simulink model "Jeos6DOF_IMU"  (R2022b)
settings: Solver=ode4  StartTime=0.0  StopTime=100  FixedStep=0.1  RelTol=1e-3
values from neighbouring files (symbols this model uses):
  a0_s2 = 0    [computeAeroForces.m]
  a0_s3 = 0    [computeAeroForces.m]
  a0_s4 = 0.05    [computeAeroForces.m]
  a0_s5 = 0.05    [computeAeroForces.m]
  AR_s2 = b_s2/c_s2    [computeSurfacePos.m]
  AR_s3 = b_s3/c_s3    [computeSurfacePos.m]
  AR_s4 = (b_s4 + b_s5)/c_s4    [computeSurfacePos.m]
  AR_s5 = (b_s4 + b_s5)/c_s5    [computeSurfacePos.m]
  area_s2 = c_s2 * b_s2    [computeSurfacePos.m]
  area_s3 = c_s3 * b_s3    [computeSurfacePos.m]
  area_s4 = c_s4 * b_s4    [computeSurfacePos.m]
  area_s5 = c_s5 * b_s5    [computeSurfacePos.m]
  c_s2 = componentMassesAndGeom(3,2)    [computeSurfacePos.m]
  c_s3 = componentMassesAndGeom(4,2)    [computeSurfacePos.m]
  c_s4 = componentMassesAndGeom(1,2)    [computeSurfacePos.m]
  c_s5 = componentMassesAndGeom(2,2)    [computeSurfacePos.m]
  CD0_s2 = 0.01    [computeAeroForces.m]
  CD0_s3 = 0.01    [computeAeroForces.m]
  CD0_s4 = 0.01    [computeAeroForces.m]
  CD0_s5 = 0.01    [computeAeroForces.m]
  CDa_s2 = 1    [computeAeroForces.m]
  CDa_s3 = 1    [computeAeroForces.m]
  CDa_s4 = 1    [computeAeroForces.m]
  CDa_s5 = 1    [computeAeroForces.m]
  CL0_s2 = 0    [computeAeroForces.m]
  CL0_s3 = 0    [computeAeroForces.m]
  CL0_s4 = 0.05    [computeAeroForces.m]
  CL0_s5 = 0.05    [computeAeroForces.m]
  CM0_s2 = 0    [computeAeroForces.m]
  CM0_s3 = 0    [computeAeroForces.m]
  CM0_s4 = -0.05    [computeAeroForces.m]
  CM0_s5 = -0.05    [computeAeroForces.m]
  CMa_s2 = 0    [computeAeroForces.m]
  CMa_s3 = 0    [computeAeroForces.m]
  CMa_s4 = 0    [computeAeroForces.m]
  CMa_s5 = 0    [computeAeroForces.m]
  e_s2 = 0.8    [computeAeroForces.m]
  e_s3 = 0.8    [computeAeroForces.m]
  e_s4 = 0.9    [computeAeroForces.m]
  e_s5 = 0.9    [computeAeroForces.m]
  i_s2 = 0    [computeAeroForces.m]
  i_s3 = 0    [computeAeroForces.m]
  i_s4 = 0.05    [computeAeroForces.m]
  i_s5 = 0.05    [computeAeroForces.m]
  Jxx = 1    [Sim_sixDOFdriverScript.m]
  Jxy = 0.    (= 0)    [Sim_sixDOFdriverScript.m]
  Jxz = 3    [Sim_sixDOFdriverScript.m]
  Jyx = 2    [Sim_sixDOFdriverScript.m]
  Jyy = 2    [Sim_sixDOFdriverScript.m]
  Jyz = 0    [Sim_sixDOFdriverScript.m]
  Jzx = Jxz    (= 3)    [Sim_sixDOFdriverScript.m]
  Jzy = Jyz    (= 0)    [Sim_sixDOFdriverScript.m]
  Jzz = 2    [Sim_sixDOFdriverScript.m]
  LL = 0.8    [Sim_sixDOFdriverScript.m]
  MM = 0.8    [Sim_sixDOFdriverScript.m]
  n_s2 = [0; 0; -1]    [computeAeroForces.m]
  n_s3 = [0; 1; 0]    [computeAeroForces.m]
  n_s4 = [0; 0; -1]    [computeAeroForces.m]
  n_s5 = [0; 0; -1]    [computeAeroForces.m]
  NN = 0.8    [Sim_sixDOFdriverScript.m]
  rEarth = 6378100    [Sim_sixDOFdriverScript.m]
  ro = 1.225    [computeAeroForces.m]
  x_S2_B_B = (x_S2_B_B_nominal + [0.25*c_s2 0 0]') - x_cg    [computeMassProps.m]
  x_S3_B_B = (x_S3_B_B_nominal + [0.25*c_s3 0 0]') - x_cg    [computeMassProps.m]
  x_S4_B_B = (x_S4_B_B_nominal + [0.25*c_s4 0 0]') - x_cg    [computeMassProps.m]
  x_S5_B_B = (x_S5_B_B_nominal + [0.25*c_s5 0 0]') - x_cg    [computeMassProps.m]
undefined symbols (not defined in the file or in its folder): earthRadius
libraries: simulink_extras x4, matrix_library x3, aerolibutil x2, sharedutil x1, simulink x1
(part 1 of 2)
settings Model: Creator=Jeo  LastModifiedBy=Jeo

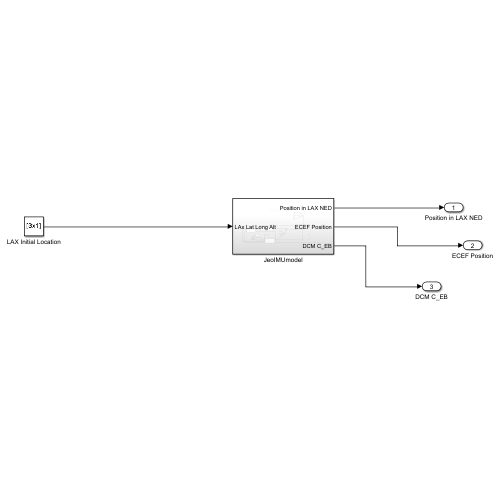
[thumbnail: Simulink's stored preview of the top-level diagram]
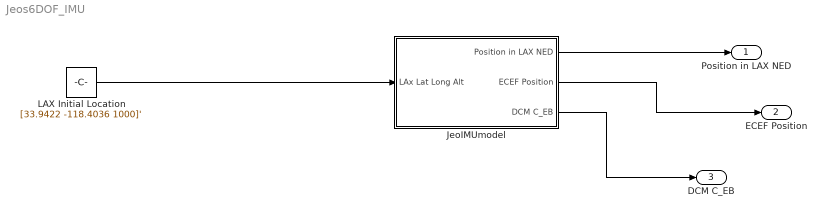
== system Jeos6DOF_IMU ==
  JeoIMUmodel : Subsystem
  LAX Initial Location : Constant  Value=[33.9422 -118.4036 1000]'
  Position in LAX NED : Outport
  ECEF Position : Outport  Port=2
  DCM C_EB : Outport  Port=3
  wires:
  LAX Initial Location/1 -> JeoIMUmodel/1(LAx Lat Long Alt)
  JeoIMUmodel/1(Position in LAX NED) -> Position in LAX NED/1
  JeoIMUmodel/2(ECEF Position) -> ECEF Position/1
  JeoIMUmodel/3(DCM C_EB) -> DCM C_EB/1

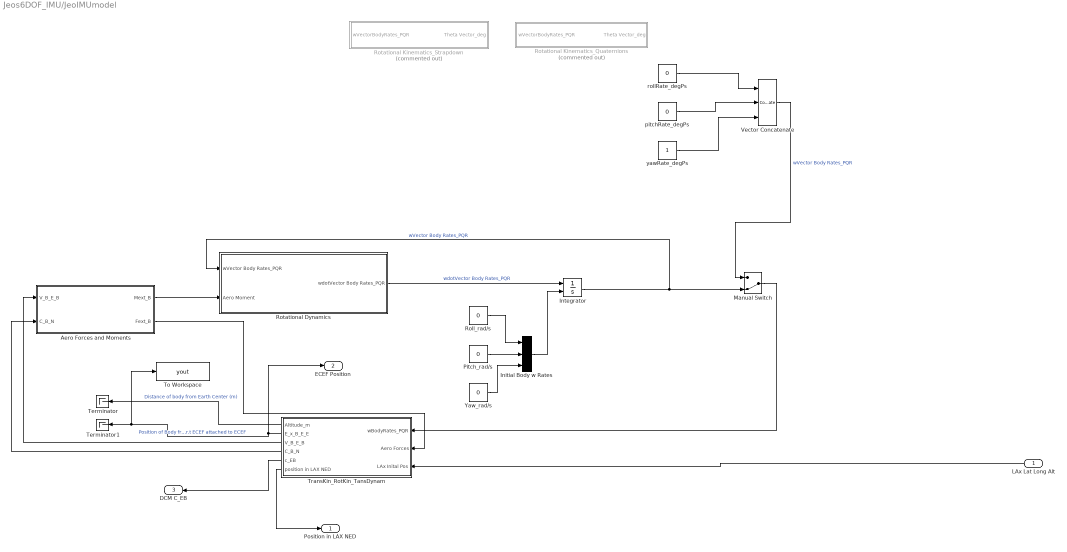
== system Jeos6DOF_IMU/JeoIMUmodel ==
  LAx Lat Long Alt : Inport
  Aero Forces and Moments : Subsystem
  Initial Body w Rates : Concatenate  NumInputs=3
  Integrator : Integrator  InitialConditionSource=external
  Manual Switch : ManualSwitch  CurrentSetting=0
  Pitch_rad/s : Constant  Value=0
  Roll_rad/s : Constant  Value=0
  Rotational Dynamics : Subsystem
  Rotational Kinematics_Quaternions : Subsystem  Commented=on
  Rotational Kinematics_Strapdown : Subsystem  Commented=on
  Terminator : Terminator
  Terminator1 : Terminator
  To Workspace : ToWorkspace  VariableName=yout  SaveFormat=Timeseries  SampleTime=-1
  TransKin_RotKin_TansDynam : Subsystem
  Vector Concatenate : Concatenate  NumInputs=3  Mode=Multidimensional array
  Yaw_rad/s : Constant  Value=0
  pitchRate_degPs : Constant  Value=0
  rollRate_degPs : Constant  Value=0
  yawRate_degPs : Constant
  Position in LAX NED : Outport
  ECEF Position : Outport  Port=2
  DCM C_EB : Outport  Port=3
  wires:
  TransKin_RotKin_TansDynam/2(E_x_B_E_E) -> Terminator1/1, To Workspace/1, ECEF Position/1  "Position of Body from ECEF w.r.t ECEF attached to ECEF"
  TransKin_RotKin_TansDynam/3(V_B_E_B) -> Aero Forces and Moments/1(V_B_E_B)
  Manual Switch/1 -> TransKin_RotKin_TansDynam/1(wBodyRates_PQR)
  TransKin_RotKin_TansDynam/1(Altitude_m) -> Terminator/1  "Distance of body from Earth Center (m)"
  Rotational Dynamics/1(wdotVector Body Rates_PQR) -> Integrator/1  "wdotVector Body Rates_PQR"
  Vector Concatenate/1 -> Manual Switch/1  "wVector Body Rates_PQR"
  TransKin_RotKin_TansDynam/4(C_B_N) -> Aero Forces and Moments/2(C_B_N)
  Integrator/1 -> Manual Switch/2, Rotational Dynamics/1(wVector Body Rates_PQR)  "wVector Body Rates_PQR"
  yawRate_degPs/1 -> Vector Concatenate/3
  Initial Body w Rates/1 -> Integrator/2
  Pitch_rad/s/1 -> Initial Body w Rates/2
  Aero Forces and Moments/1(Mext_B) -> Rotational Dynamics/2(Aero Moment)
  LAx Lat Long Alt/1 -> TransKin_RotKin_TansDynam/3(LAx Inital Pos)
  Roll_rad/s/1 -> Initial Body w Rates/1
  Aero Forces and Moments/2(Fext_B) -> TransKin_RotKin_TansDynam/2(Aero Forces)
  Yaw_rad/s/1 -> Initial Body w Rates/3
  rollRate_degPs/1 -> Vector Concatenate/1
  pitchRate_degPs/1 -> Vector Concatenate/2
  TransKin_RotKin_TansDynam/5(c_EB) -> DCM C_EB/1
  TransKin_RotKin_TansDynam/6(position in LAX NED) -> Position in LAX NED/1

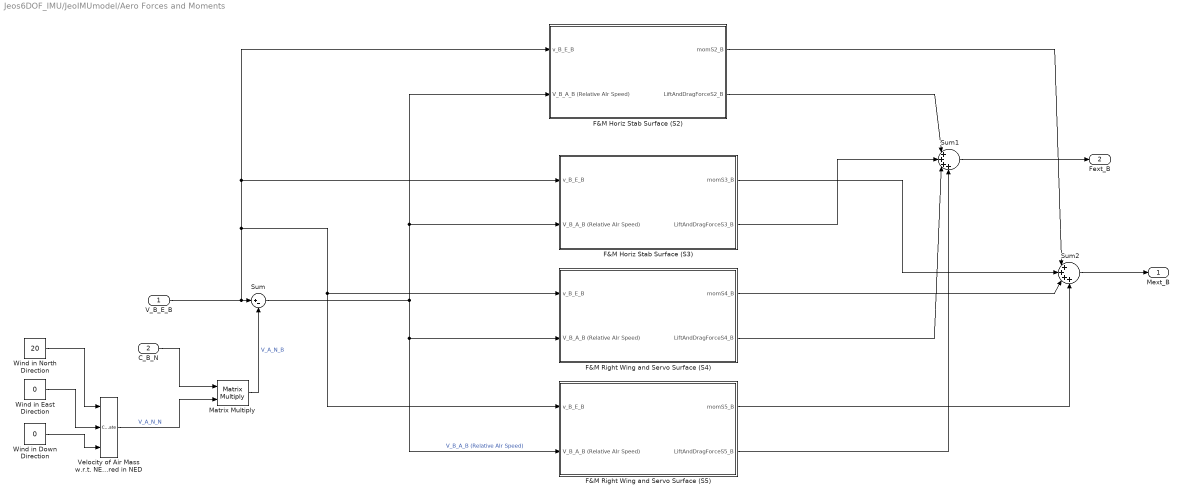
== system Jeos6DOF_IMU/JeoIMUmodel/Aero Forces and Moments ==
  V_B_E_B : Inport
  C_B_N : Inport  Port=2
  F&M Horiz Stab Surface (S2) : Subsystem
  F&M Horiz Stab Surface (S3) : Subsystem
  F&M Right Wing and Servo Surface (S4) : Subsystem
  F&M Right Wing and Servo Surface (S5) : Subsystem
  Matrix Multiply : Product  Multiplication=Matrix(*)
  Sum : Sum  Inputs=|+-
  Sum1 : Sum  Inputs=|++++
  Sum2 : Sum  Inputs=|++++
  Velocity of Air Mass w.r.t. NED as measured in NED : Concatenate  NumInputs=3
  Wind in Down Direction : Constant  Value=0
  Wind in East Direction : Constant  Value=0
  Wind in North Direction : Constant  Value=20
  Mext_B : Outport
  Fext_B : Outport  Port=2
  wires:
  V_B_E_B/1 -> F&M Right Wing and Servo Surface (S5)/1(v_B_E_B), F&M Right Wing and Servo Surface (S4)/1(v_B_E_B), F&M Horiz Stab Surface (S2)/1(v_B_E_B), F&M Horiz Stab Surface (S3)/1(v_B_E_B), Sum/1
  Velocity of Air Mass w.r.t. NED as measured in NED/1 -> Matrix Multiply/2  "V_A_N_N"
  Wind in North Direction/1 -> Velocity of Air Mass w.r.t. NED as measured in NED/1
  Wind in East Direction/1 -> Velocity of Air Mass w.r.t. NED as measured in NED/2
  Wind in Down Direction/1 -> Velocity of Air Mass w.r.t. NED as measured in NED/3
  Sum/1 -> F&M Horiz Stab Surface (S2)/2(V_B_A_B (Relative AIr Speed)), F&M Horiz Stab Surface (S3)/2(V_B_A_B (Relative AIr Speed)), F&M Right Wing and Servo Surface (S5)/2(V_B_A_B (Relative AIr Speed)), F&M Right Wing and Servo Surface (S4)/2(V_B_A_B (Relative AIr Speed))  "V_B_A_B (Relative AIr Speed)"
  F&M Horiz Stab Surface (S2)/2(LiftAndDragForceS2_B) -> Sum1/1
  F&M Horiz Stab Surface (S3)/2(LiftAndDragForceS3_B) -> Sum1/2
  F&M Right Wing and Servo Surface (S4)/2(LiftAndDragForceS4_B) -> Sum1/3
  F&M Right Wing and Servo Surface (S5)/2(LiftAndDragForceS5_B) -> Sum1/4
  Sum1/1 -> Fext_B/1
  F&M Horiz Stab Surface (S2)/1(momS2_B) -> Sum2/1
  F&M Horiz Stab Surface (S3)/1(momS3_B) -> Sum2/2
  F&M Right Wing and Servo Surface (S4)/1(momS4_B) -> Sum2/3
  F&M Right Wing and Servo Surface (S5)/1(momS5_B) -> Sum2/4
  Sum2/1 -> Mext_B/1
  C_B_N/1 -> Matrix Multiply/1
  Matrix Multiply/1 -> Sum/2  "V_A_N_B"

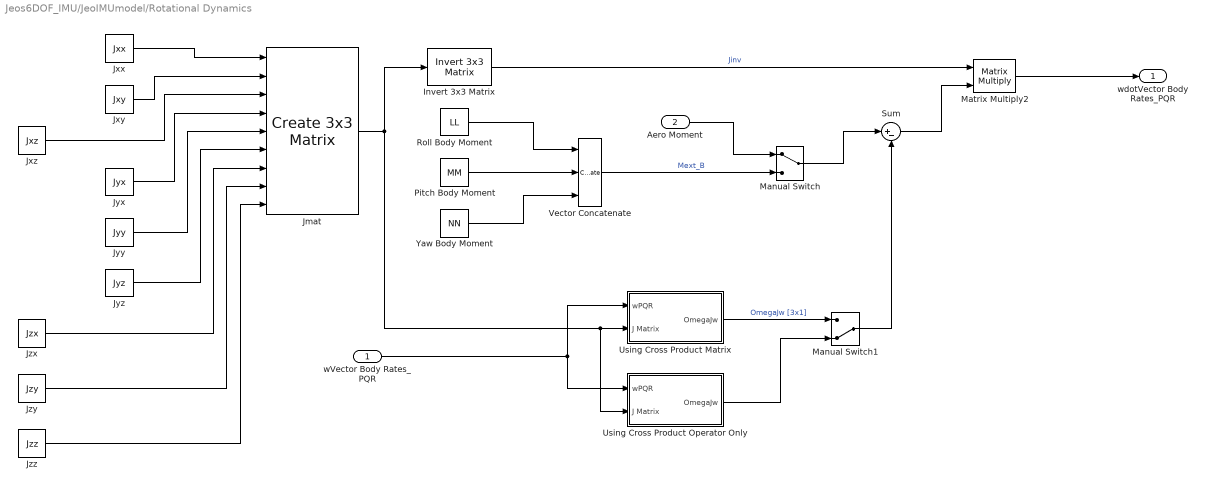
== system Jeos6DOF_IMU/JeoIMUmodel/Rotational Dynamics ==
  wVector Body Rates_PQR : Inport
  Aero Moment : Inport  Port=2
  Invert 3x3 Matrix : aerolibutil/Invert  3x3 Matrix
  Jmat : sharedutil/Create 3x3 Matrix  aMode=aMode
      settings: LibrarySourceBlock=aerolibutil/Create 3x3 Matrix
  Jxx : Constant  Value=Jxx
  Jxy : Constant  Value=Jxy
  Jxz : Constant  Value=Jxz
  Jyx : Constant  Value=Jyx
  Jyy : Constant  Value=Jyy
  Jyz : Constant  Value=Jyz
  Jzx : Constant  Value=Jzx
  Jzy : Constant  Value=Jzy
  Jzz : Constant  Value=Jzz
  Manual Switch : ManualSwitch
  Manual Switch1 : ManualSwitch  CurrentSetting=0
  Matrix Multiply2 : Product  Multiplication=Matrix(*)
  Pitch Body Moment : Constant  Value=MM
  Roll Body Moment : Constant  Value=LL
  Sum : Sum  Inputs=|+-
  Using Cross Product Matrix : Subsystem
  Using Cross Product Operator Only : Subsystem
  Vector Concatenate : Concatenate  NumInputs=3
  Yaw Body Moment : Constant  Value=NN
  wdotVector Body Rates_PQR : Outport
  wires:
  wVector Body Rates_PQR/1 -> Using Cross Product Operator Only/1(wPQR), Using Cross Product Matrix/1(wPQR)
  Jmat/1 -> Using Cross Product Matrix/2(J Matrix), Using Cross Product Operator Only/2(J Matrix), Invert 3x3 Matrix/1
  Using Cross Product Matrix/1(OmegaJw) -> Manual Switch1/1  "OmegaJw [3x1]"
  Sum/1 -> Matrix Multiply2/2
  Matrix Multiply2/1 -> wdotVector Body Rates_PQR/1
  Jxx/1 -> Jmat/1
  Jxy/1 -> Jmat/2
  Jxz/1 -> Jmat/3
  Jyx/1 -> Jmat/4
  Jyy/1 -> Jmat/5
  Jyz/1 -> Jmat/6
  Jzx/1 -> Jmat/7
  Jzy/1 -> Jmat/8
  Jzz/1 -> Jmat/9
  Invert 3x3 Matrix/1 -> Matrix Multiply2/1  "Jinv"
  Roll Body Moment/1 -> Vector Concatenate/1
  Pitch Body Moment/1 -> Vector Concatenate/2
  Yaw Body Moment/1 -> Vector Concatenate/3
  Vector Concatenate/1 -> Manual Switch/2  "Mext_B"
  Aero Moment/1 -> Manual Switch/1
  Manual Switch/1 -> Sum/1
  Manual Switch1/1 -> Sum/2
  Using Cross Product Operator Only/1(OmegaJw) -> Manual Switch1/2

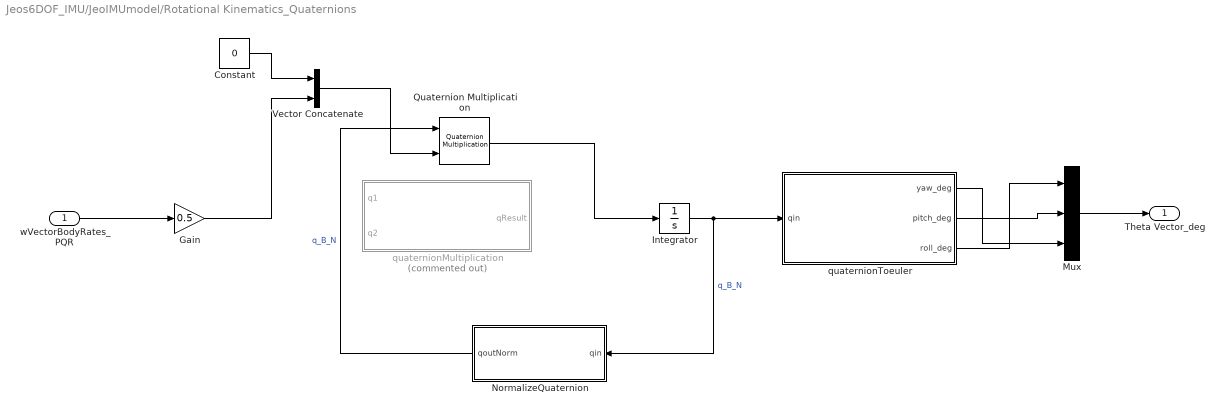
== system Jeos6DOF_IMU/JeoIMUmodel/Rotational Kinematics_Quaternions ==
  wVectorBodyRates_PQR : Inport
  Constant : Constant  Value=0
  Gain : Gain  Gain=0.5
  Integrator : Integrator
  Mux : Mux  Inputs=3
  NormalizeQuaternion : MATLAB Function  TreatAsAtomicUnit=on
  Quaternion Multiplication : aerolibutil/Quaternion Multiplication
  Vector Concatenate : Concatenate
  quaternionMultiplication : MATLAB Function  Commented=on  TreatAsAtomicUnit=on
  quaternionToeuler : MATLAB Function  TreatAsAtomicUnit=on
  Theta Vector_deg : Outport
  wires:
  wVectorBodyRates_PQR/1 -> Gain/1
  Gain/1 -> Vector Concatenate/2
  Constant/1 -> Vector Concatenate/1
  Integrator/1 -> NormalizeQuaternion/1(qin), quaternionToeuler/1(qin)  "q_B_N"
  quaternionToeuler/3(roll_deg) -> Mux/1
  quaternionToeuler/2(pitch_deg) -> Mux/2
  quaternionToeuler/1(yaw_deg) -> Mux/3
  NormalizeQuaternion/1(qoutNorm) -> Quaternion Multiplication/1  "q_B_N"
  Mux/1 -> Theta Vector_deg/1
  Quaternion Multiplication/1 -> Integrator/1
  Vector Concatenate/1 -> Quaternion Multiplication/2

== system Jeos6DOF_IMU/JeoIMUmodel/Rotational Kinematics_Strapdown ==
  wVectorBodyRates_PQR : Inport
  Demux : Demux  Outputs=3
  Integrator : Integrator
  MatrixMultiply : Product  Multiplication=Matrix(*)
  Mux : Mux  Inputs=3
  Omega_B_N : MATLAB Function  TreatAsAtomicUnit=on
  dcmTOeuler : MATLAB Function  TreatAsAtomicUnit=on
  Theta Vector_deg : Outport
  wires:
  wVectorBodyRates_PQR/1 -> Demux/1
  Demux/1 -> Omega_B_N/1(P_degPs)
  Demux/2 -> Omega_B_N/2(Q_degPs)
  Demux/3 -> Omega_B_N/3(R_degPs)
  Omega_B_N/1(y) -> MatrixMultiply/1  "omega_B_N"
  MatrixMultiply/1 -> Integrator/1  "cdot_N_B"
  Integrator/1 -> MatrixMultiply/2, dcmTOeuler/1(inputDCM)  "c_N_B"
  dcmTOeuler/3(roll_deg) -> Mux/1
  dcmTOeuler/2(pitch_deg) -> Mux/2
  dcmTOeuler/1(yaw_deg) -> Mux/3
  Mux/1 -> Theta Vector_deg/1  "Theta Vector_deg"

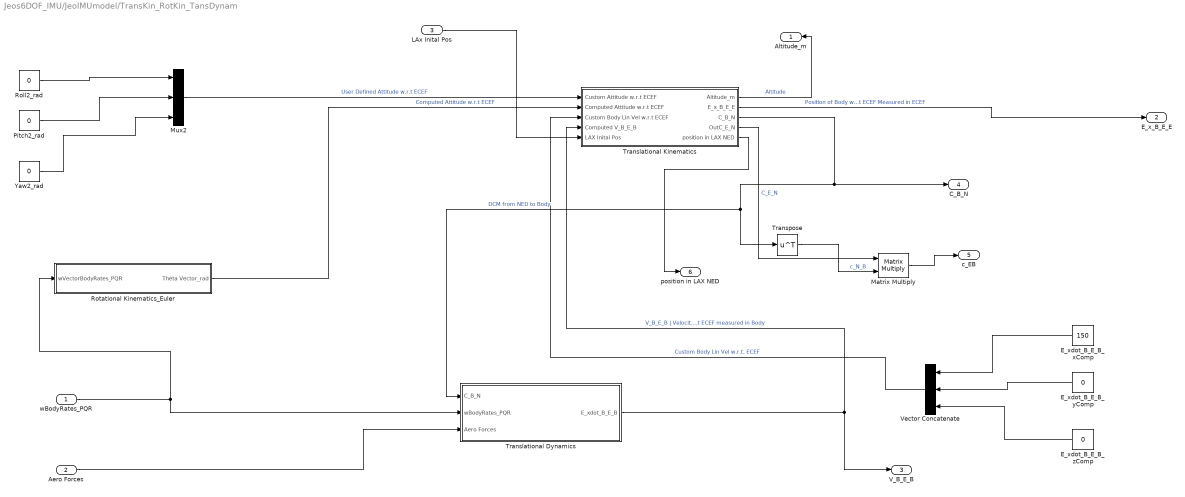
== system Jeos6DOF_IMU/JeoIMUmodel/TransKin_RotKin_TansDynam ==
  wBodyRates_PQR : Inport
  Aero Forces : Inport  Port=2
  LAx Inital Pos : Inport  Port=3
  E_xdot_B_E_B_xComp : Constant  Value=150
  E_xdot_B_E_B_yComp : Constant  Value=0
  E_xdot_B_E_B_zComp : Constant  Value=0
  Matrix Multiply : Product  Multiplication=Matrix(*)
  Mux2 : Mux  Inputs=3
  Pitch2_rad : Constant  Value=0
  Roll2_rad : Constant  Value=0
  Rotational Kinematics_Euler : Subsystem
  Translational Dynamics : Subsystem
  Translational Kinematics : Subsystem
  Transpose : Math  Operator=transpose
  Vector Concatenate : Concatenate  NumInputs=3
  Yaw2_rad : Constant  Value=0
  Altitude_m : Outport
  E_x_B_E_E : Outport  Port=2
  V_B_E_B : Outport  Port=3
  C_B_N : Outport  Port=4
  c_EB : Outport  Port=5
  position in LAX NED : Outport  Port=6
  wires:
  Pitch2_rad/1 -> Mux2/2
  Translational Dynamics/1(E_xdot_B_E_B) -> Translational Kinematics/4(Computed V_B_E_B), V_B_E_B/1  "V_B_E_B | Velocity of Body w.r.t ECEF measured in Body"
  wBodyRates_PQR/1 -> Translational Dynamics/2(wBodyRates_PQR), Rotational Kinematics_Euler/1(wVectorBodyRates_PQR)
  Roll2_rad/1 -> Mux2/1
  Yaw2_rad/1 -> Mux2/3
  E_xdot_B_E_B_xComp/1 -> Vector Concatenate/1
  E_xdot_B_E_B_yComp/1 -> Vector Concatenate/2
  E_xdot_B_E_B_zComp/1 -> Vector Concatenate/3
  Aero Forces/1 -> Translational Dynamics/3(Aero Forces)
  Mux2/1 -> Translational Kinematics/1(Custom Attitude w.r.t ECEF)  "User Defined Attitude w.r.t ECEF"
  Rotational Kinematics_Euler/1(Theta Vector_rad) -> Translational Kinematics/2(Computed Attitude w.r.t ECEF)  "Computed Attitude w.r.t ECEF"
  Vector Concatenate/1 -> Translational Kinematics/3(Custom Body Lin Vel w.r.t ECEF)  "Custom Body Lin Vel w.r.t. ECEF"
  Translational Kinematics/1(Altitude_m) -> Altitude_m/1  "Altitude"
  Translational Kinematics/2(E_x_B_E_E) -> E_x_B_E_E/1  "Position of Body w.r.t ECEF Measured in ECEF"
  Translational Kinematics/3(C_B_N) -> Transpose/1, Translational Dynamics/1(C_B_N), C_B_N/1  "DCM from NED to Body"
  LAx Inital Pos/1 -> Translational Kinematics/5(LAX Inital Pos)
  Matrix Multiply/1 -> c_EB/1
  Transpose/1 -> Matrix Multiply/2  "c_N_B"
  Translational Kinematics/4(OutC_E_N) -> Matrix Multiply/1  "C_E_N"
  Translational Kinematics/5(position in LAX NED) -> position in LAX NED/1

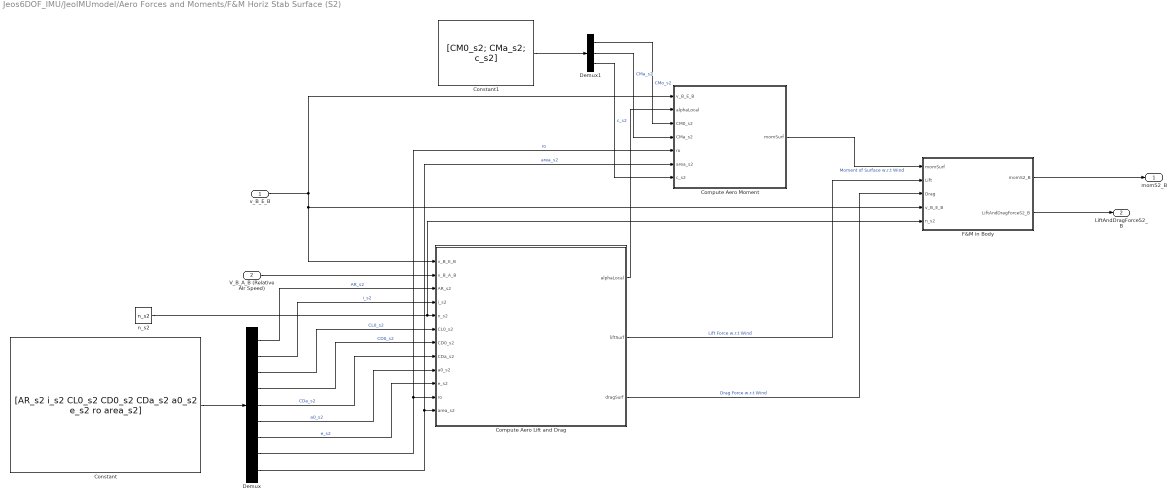
== system Jeos6DOF_IMU/JeoIMUmodel/Aero Forces and Moments/F&M Horiz Stab Surface (S2) ==
  v_B_E_B : Inport
  V_B_A_B (Relative AIr Speed) : Inport  Port=2
  Compute Aero Lift and Drag : MATLAB Function  TreatAsAtomicUnit=on
  Compute Aero Moment : MATLAB Function  TreatAsAtomicUnit=on
  Constant : Constant  Value=[AR_s2 i_s2 CL0_s2 CD0_s2 CDa_s2 a0_s2 e_s2 ro area_s2]
  Constant1 : Constant  Value=[CM0_s2; CMa_s2; c_s2]
  Demux : Demux  Outputs=9
  Demux1 : Demux  Outputs=3
  F&M in Body : Subsystem
  n_s2 : Constant  Value=n_s2
  momS2_B : Outport
  LiftAndDragForceS2_B : Outport  Port=2
  wires:
  Compute Aero Lift and Drag/2(liftSurf) -> F&M in Body/2(Lift)  "Lift Force w.r.t Wind"
  Compute Aero Moment/1(momSurf) -> F&M in Body/1(momSurf)  "Moment of Surface w.r.t Wind"
  Compute Aero Lift and Drag/3(dragSurf) -> F&M in Body/3(Drag)  "Drag Force w.r.t Wind"
  F&M in Body/2(LiftAndDragForceS2_B) -> LiftAndDragForceS2_B/1
  Compute Aero Lift and Drag/1(alphaLocal) -> Compute Aero Moment/2(alphaLocal)
  v_B_E_B/1 -> Compute Aero Lift and Drag/1(v_B_E_B), F&M in Body/4(v_B_E_B), Compute Aero Moment/1(v_B_E_B)
  F&M in Body/1(momS2_B) -> momS2_B/1
  V_B_A_B (Relative AIr Speed)/1 -> Compute Aero Lift and Drag/2(v_B_A_B)
  Constant/1 -> Demux/1
  Demux/1 -> Compute Aero Lift and Drag/3(AR_s2)  "AR_s2"
  Demux/2 -> Compute Aero Lift and Drag/4(i_s2)  "i_s2"
  Demux/3 -> Compute Aero Lift and Drag/6(CL0_s2)  "CL0_s2"
  Demux/4 -> Compute Aero Lift and Drag/7(CD0_s2)  "CD0_s2"
  Demux/5 -> Compute Aero Lift and Drag/8(CDa_s2)  "CDa_s2"
  Demux/6 -> Compute Aero Lift and Drag/9(a0_s2)  "a0_s2"
  Demux/7 -> Compute Aero Lift and Drag/10(e_s2)  "e_s2"
  Demux/8 -> Compute Aero Moment/5(ro), Compute Aero Lift and Drag/11(ro)  "ro"
  Demux/9 -> Compute Aero Moment/6(area_s2), Compute Aero Lift and Drag/12(area_s2)  "area_s2"
  Constant1/1 -> Demux1/1
  Demux1/1 -> Compute Aero Moment/3(CM0_s2)  "CMo_s2"
  Demux1/2 -> Compute Aero Moment/4(CMa_s2)  "CMa_s2"
  Demux1/3 -> Compute Aero Moment/7(c_s2)  "c_s2"
  n_s2/1 -> F&M in Body/5(n_s2), Compute Aero Lift and Drag/5(n_s2)

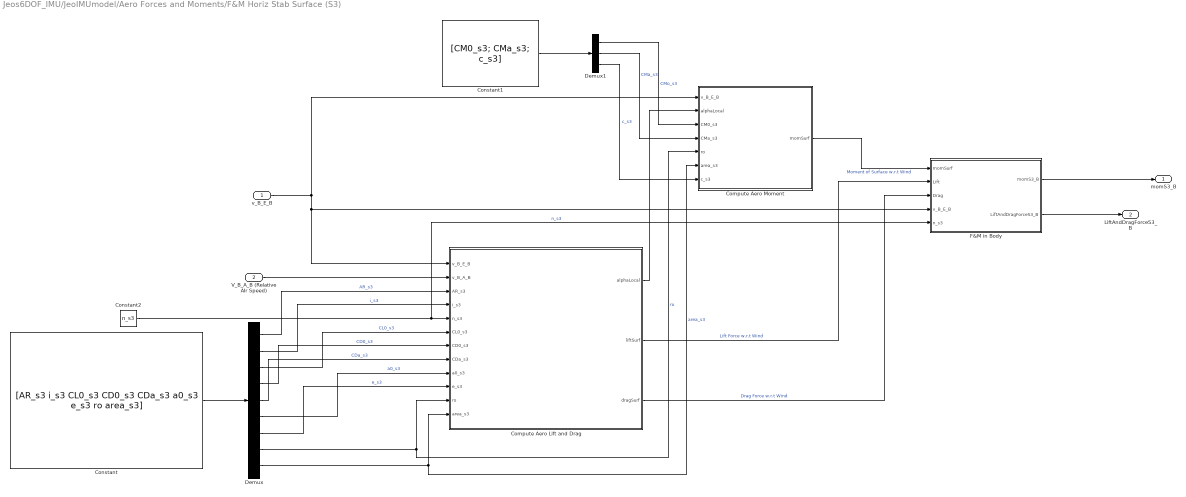
== system Jeos6DOF_IMU/JeoIMUmodel/Aero Forces and Moments/F&M Horiz Stab Surface (S3) ==
  v_B_E_B : Inport
  V_B_A_B (Relative AIr Speed) : Inport  Port=2
  Compute Aero Lift and Drag : MATLAB Function  TreatAsAtomicUnit=on
  Compute Aero Moment : MATLAB Function  TreatAsAtomicUnit=on
  Constant : Constant  Value=[AR_s3 i_s3 CL0_s3 CD0_s3 CDa_s3 a0_s3 e_s3 ro area_s3]
  Constant1 : Constant  Value=[CM0_s3; CMa_s3; c_s3]
  Constant2 : Constant  Value=n_s3
  Demux : Demux  Outputs=9
  Demux1 : Demux  Outputs=3
  F&M in Body : Subsystem
  momS3_B : Outport
  LiftAndDragForceS3_B : Outport  Port=2
  wires:
  Compute Aero Lift and Drag/2(liftSurf) -> F&M in Body/2(Lift)  "Lift Force w.r.t Wind"
  Compute Aero Moment/1(momSurf) -> F&M in Body/1(momSurf)  "Moment of Surface w.r.t Wind"
  Compute Aero Lift and Drag/3(dragSurf) -> F&M in Body/3(Drag)  "Drag Force w.r.t Wind"
  F&M in Body/2(LiftAndDragForceS3_B) -> LiftAndDragForceS3_B/1
  Compute Aero Lift and Drag/1(alphaLocal) -> Compute Aero Moment/2(alphaLocal)
  v_B_E_B/1 -> Compute Aero Lift and Drag/1(v_B_E_B), F&M in Body/4(v_B_E_B), Compute Aero Moment/1(v_B_E_B)
  F&M in Body/1(momS3_B) -> momS3_B/1
  V_B_A_B (Relative AIr Speed)/1 -> Compute Aero Lift and Drag/2(v_B_A_B)
  Constant/1 -> Demux/1
  Demux/1 -> Compute Aero Lift and Drag/3(AR_s3)  "AR_s3"
  Demux/2 -> Compute Aero Lift and Drag/4(i_s3)  "i_s3"
  Constant2/1 -> F&M in Body/5(n_s3), Compute Aero Lift and Drag/5(n_s3)  "n_s3"
  Demux/3 -> Compute Aero Lift and Drag/6(CL0_s3)  "CL0_s3"
  Demux/4 -> Compute Aero Lift and Drag/7(CD0_s3)  "CD0_s3"
  Demux/5 -> Compute Aero Lift and Drag/8(CDa_s3)  "CDa_s3"
  Demux/6 -> Compute Aero Lift and Drag/9(a0_s3)  "a0_s3"
  Demux/7 -> Compute Aero Lift and Drag/10(e_s3)  "e_s3"
  Demux/8 -> Compute Aero Moment/5(ro), Compute Aero Lift and Drag/11(ro)  "ro"
  Demux/9 -> Compute Aero Moment/6(area_s3), Compute Aero Lift and Drag/12(area_s3)  "area_s3"
  Constant1/1 -> Demux1/1
  Demux1/1 -> Compute Aero Moment/3(CM0_s3)  "CMo_s3"
  Demux1/2 -> Compute Aero Moment/4(CMa_s3)  "CMa_s3"
  Demux1/3 -> Compute Aero Moment/7(c_s3)  "c_s3"

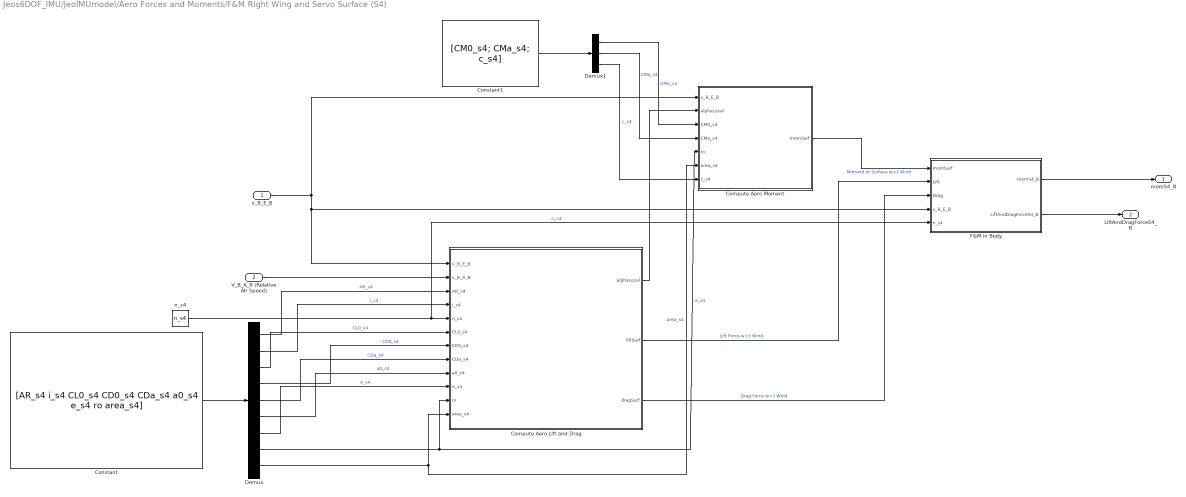
== system Jeos6DOF_IMU/JeoIMUmodel/Aero Forces and Moments/F&M Right Wing and Servo Surface (S4) ==
  v_B_E_B : Inport
  V_B_A_B (Relative AIr Speed) : Inport  Port=2
  Compute Aero Lift and Drag : MATLAB Function  TreatAsAtomicUnit=on
  Compute Aero Moment : MATLAB Function  TreatAsAtomicUnit=on
  Constant : Constant  Value="[AR_s4 i_s4  CL0_s4 CD0_s4 CDa_s4 a0_s4 e_s4 ro area_s4]"
  Constant1 : Constant  Value=[CM0_s4; CMa_s4; c_s4]
  Demux : Demux  Outputs=9
  Demux1 : Demux  Outputs=3
  F&M in Body : Subsystem
  n_s4 : Constant  Value=n_s4
  momS4_B : Outport
  LiftAndDragForceS4_B : Outport  Port=2
  wires:
  Compute Aero Lift and Drag/2(liftSurf) -> F&M in Body/2(Lift)  "Lift Force w.r.t Wind"
  Compute Aero Moment/1(momSurf) -> F&M in Body/1(momSurf)  "Moment of Surface w.r.t Wind"
  Compute Aero Lift and Drag/3(dragSurf) -> F&M in Body/3(Drag)  "Drag Force w.r.t Wind"
  F&M in Body/2(LiftAndDragForceS4_B) -> LiftAndDragForceS4_B/1
  Compute Aero Lift and Drag/1(alphaLocal) -> Compute Aero Moment/2(alphaLocal)
  v_B_E_B/1 -> Compute Aero Lift and Drag/1(v_B_E_B), F&M in Body/4(v_B_E_B), Compute Aero Moment/1(v_B_E_B)
  F&M in Body/1(momS4_B) -> momS4_B/1
  V_B_A_B (Relative AIr Speed)/1 -> Compute Aero Lift and Drag/2(v_B_A_B)
  Constant/1 -> Demux/1
  Demux/1 -> Compute Aero Lift and Drag/3(AR_s4)  "AR_s4"
  Demux/2 -> Compute Aero Lift and Drag/4(i_s4)  "i_s4"
  n_s4/1 -> F&M in Body/5(n_s4), Compute Aero Lift and Drag/5(n_s4)  "n_s4"
  Demux/3 -> Compute Aero Lift and Drag/6(CL0_s4)  "CL0_s4"
  Demux/4 -> Compute Aero Lift and Drag/7(CD0_s4)  "CD0_s4"
  Demux/5 -> Compute Aero Lift and Drag/8(CDa_s4)  "CDa_s4"
  Demux/6 -> Compute Aero Lift and Drag/9(a0_s4)  "a0_s4"
  Demux/7 -> Compute Aero Lift and Drag/10(e_s4)  "e_s4"
  Demux/9 -> Compute Aero Moment/6(area_s4), Compute Aero Lift and Drag/12(area_s4)  "area_s4"
  Constant1/1 -> Demux1/1
  Demux1/1 -> Compute Aero Moment/3(CM0_s4)  "CMo_s4"
  Demux1/2 -> Compute Aero Moment/4(CMa_s4)  "CMa_s4"
  Demux1/3 -> Compute Aero Moment/7(c_s4)  "c_s4"
  Demux/8 -> Compute Aero Moment/5(ro), Compute Aero Lift and Drag/11(ro)  "e_s4"

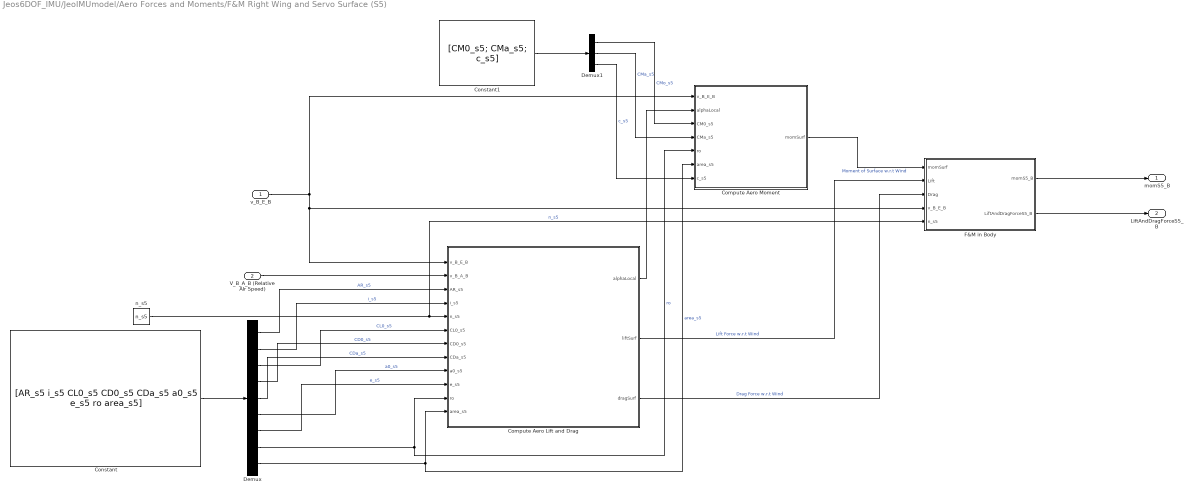
== system Jeos6DOF_IMU/JeoIMUmodel/Aero Forces and Moments/F&M Right Wing and Servo Surface (S5) ==
  v_B_E_B : Inport
  V_B_A_B (Relative AIr Speed) : Inport  Port=2
  Compute Aero Lift and Drag : MATLAB Function  TreatAsAtomicUnit=on
  Compute Aero Moment : MATLAB Function  TreatAsAtomicUnit=on
  Constant : Constant  Value=[AR_s5 i_s5 CL0_s5 CD0_s5 CDa_s5 a0_s5 e_s5 ro area_s5]
  Constant1 : Constant  Value=[CM0_s5; CMa_s5; c_s5]
  Demux : Demux  Outputs=9
  Demux1 : Demux  Outputs=3
  F&M in Body : Subsystem
  n_s5 : Constant  Value=n_s5
  momS5_B : Outport
  LiftAndDragForceS5_B : Outport  Port=2
  wires:
  Compute Aero Lift and Drag/2(liftSurf) -> F&M in Body/2(Lift)  "Lift Force w.r.t Wind"
  Compute Aero Moment/1(momSurf) -> F&M in Body/1(momSurf)  "Moment of Surface w.r.t Wind"
  Compute Aero Lift and Drag/3(dragSurf) -> F&M in Body/3(Drag)  "Drag Force w.r.t Wind"
  F&M in Body/2(LiftAndDragForceS5_B) -> LiftAndDragForceS5_B/1
  Compute Aero Lift and Drag/1(alphaLocal) -> Compute Aero Moment/2(alphaLocal)
  v_B_E_B/1 -> Compute Aero Lift and Drag/1(v_B_E_B), F&M in Body/4(v_B_E_B), Compute Aero Moment/1(v_B_E_B)
  F&M in Body/1(momS5_B) -> momS5_B/1
  V_B_A_B (Relative AIr Speed)/1 -> Compute Aero Lift and Drag/2(v_B_A_B)
  Constant/1 -> Demux/1
  Demux/1 -> Compute Aero Lift and Drag/3(AR_s5)  "AR_s5"
  Demux/2 -> Compute Aero Lift and Drag/4(i_s5)  "i_s5"
  n_s5/1 -> F&M in Body/5(n_s5), Compute Aero Lift and Drag/5(n_s5)  "n_s5"
  Demux/3 -> Compute Aero Lift and Drag/6(CL0_s5)  "CL0_s5"
  Demux/4 -> Compute Aero Lift and Drag/7(CD0_s5)  "CD0_s5"
  Demux/5 -> Compute Aero Lift and Drag/8(CDa_s5)  "CDa_s5"
  Demux/6 -> Compute Aero Lift and Drag/9(a0_s5)  "a0_s5"
  Demux/7 -> Compute Aero Lift and Drag/10(e_s5)  "e_s5"
  Demux/8 -> Compute Aero Moment/5(ro), Compute Aero Lift and Drag/11(ro)  "ro"
  Demux/9 -> Compute Aero Moment/6(area_s5), Compute Aero Lift and Drag/12(area_s5)  "area_s5"
  Constant1/1 -> Demux1/1
  Demux1/1 -> Compute Aero Moment/3(CM0_s5)  "CMo_s5"
  Demux1/2 -> Compute Aero Moment/4(CMa_s5)  "CMa_s5"
  Demux1/3 -> Compute Aero Moment/7(c_s5)  "c_s5"

== system Jeos6DOF_IMU/JeoIMUmodel/Rotational Dynamics/Using Cross Product Matrix ==
  wPQR : Inport
  J Matrix : Inport  Port=2
  Matrix Multiply : Product  Multiplication=Matrix(*)
  Matrix Multiply1 : Product  Multiplication=Matrix(*)
  Omega Cross Matrix : MATLAB Function  TreatAsAtomicUnit=on
  OmegaJw : Outport
  wires:
  wPQR/1 -> Omega Cross Matrix/1(PQR), Matrix Multiply1/2
  J Matrix/1 -> Matrix Multiply1/1
  Omega Cross Matrix/1(omegaMat) -> Matrix Multiply/1
  Matrix Multiply1/1 -> Matrix Multiply/2  "Jw"
  Matrix Multiply/1 -> OmegaJw/1

== system Jeos6DOF_IMU/JeoIMUmodel/Rotational Dynamics/Using Cross Product Operator Only ==
  wPQR : Inport
  J Matrix : Inport  Port=2
  Cross Product : matrix_library/Cross Product
  Matrix Multiply1 : Product  Multiplication=Matrix(*)
  OmegaJw : Outport
  wires:
  wPQR/1 -> Matrix Multiply1/2, Cross Product/1
  J Matrix/1 -> Matrix Multiply1/1
  Matrix Multiply1/1 -> Cross Product/2  "Jw"
  Cross Product/1 -> OmegaJw/1

== system Jeos6DOF_IMU/JeoIMUmodel/TransKin_RotKin_TansDynam/Rotational Kinematics_Euler ==
  wVectorBodyRates_PQR : Inport
  Demux : Demux  Outputs=3
  HinvMatrix : MATLAB Function  TreatAsAtomicUnit=on
  Initial Attitude_rad w.r.t ECEF : Constant  Value=[0; 0; 0]
  Integrator : Integrator  InitialConditionSource=external  InitialCondition=[0;30;30]
  MatrixMultiply : Product  Multiplication=Matrix(*)
  Scope : Scope
  Terminator : Terminator
  Theta Vector_rad : Outport
  wires:
  HinvMatrix/1(hinv) -> MatrixMultiply/1
  MatrixMultiply/1 -> Integrator/1  "Theta Vector Dot"
  Integrator/1 -> Demux/1, Theta Vector_rad/1, Scope/1  "Theta Vector_rad"
  Demux/1 -> HinvMatrix/2(rollPhi)  "roll_rad"
  Demux/2 -> HinvMatrix/1(pitchTheta)  "pitch_rad"
  Demux/3 -> Terminator/1  "yaw_rad"
  wVectorBodyRates_PQR/1 -> MatrixMultiply/2  "wVector Body Rates_PQR"
  Initial Attitude_rad w.r.t ECEF/1 -> Integrator/2

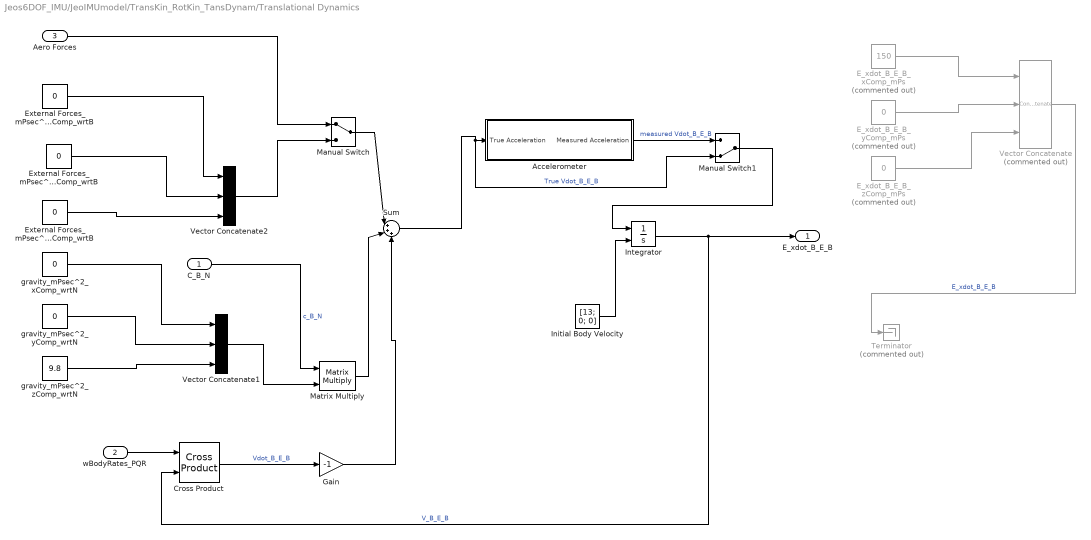
== system Jeos6DOF_IMU/JeoIMUmodel/TransKin_RotKin_TansDynam/Translational Dynamics ==
  C_B_N : Inport
  wBodyRates_PQR : Inport  Port=2
  Aero Forces : Inport  Port=3
  Accelerometer : Subsystem
  Cross Product : matrix_library/Cross Product
  E_xdot_B_E_B_xComp_mPs : Constant  Commented=on  Value=150
  E_xdot_B_E_B_yComp_mPs : Constant  Commented=on  Value=0
  E_xdot_B_E_B_zComp_mPs : Constant  Commented=on  Value=0
  External Forces_mPsec^2_xComp_wrtB : Constant  Value=0
  External Forces_mPsec^2_yComp_wrtB : Constant  Value=0
  External Forces_mPsec^2_zComp_wrtB : Constant  Value=0
  Gain : Gain  Gain=-1
  Initial Body Velocity : Constant  Value=[13; 0; 0]
  Integrator : Integrator  InitialConditionSource=external  InitialCondition=[50;0;0]
  Manual Switch : ManualSwitch
  Manual Switch1 : ManualSwitch  CurrentSetting=0
  Matrix Multiply : Product  Multiplication=Matrix(*)
  Sum : Sum  Inputs=|+++
  Terminator : Terminator  Commented=on
  Vector Concatenate : Concatenate  Commented=on  NumInputs=3  Mode=Multidimensional array
  Vector Concatenate1 : Concatenate  NumInputs=3
  Vector Concatenate2 : Concatenate  NumInputs=3
  gravity_mPsec^2_xComp_wrtN : Constant  Value=0
  gravity_mPsec^2_yComp_wrtN : Constant  Value=0
  gravity_mPsec^2_zComp_wrtN : Constant  Value=9.8
  E_xdot_B_E_B : Outport
  wires:
  E_xdot_B_E_B_xComp_mPs/1 -> Vector Concatenate/1
  E_xdot_B_E_B_zComp_mPs/1 -> Vector Concatenate/3
  E_xdot_B_E_B_yComp_mPs/1 -> Vector Concatenate/2
  Vector Concatenate/1 -> Terminator/1  "E_xdot_B_E_B"
  External Forces_mPsec^2_xComp_wrtB/1 -> Vector Concatenate2/1
  gravity_mPsec^2_xComp_wrtN/1 -> Vector Concatenate1/1
  wBodyRates_PQR/1 -> Cross Product/1
  Cross Product/1 -> Gain/1  "Vdot_B_E_B"
  Integrator/1 -> E_xdot_B_E_B/1, Cross Product/2  "V_B_E_B"
  Gain/1 -> Sum/3
  Sum/1 -> Manual Switch1/2, Accelerometer/1(True Acceleration)  "True Vdot_B_E_B"
  gravity_mPsec^2_yComp_wrtN/1 -> Vector Concatenate1/2
  gravity_mPsec^2_zComp_wrtN/1 -> Vector Concatenate1/3
  Vector Concatenate1/1 -> Matrix Multiply/2
  External Forces_mPsec^2_yComp_wrtB/1 -> Vector Concatenate2/2
  External Forces_mPsec^2_zComp_wrtB/1 -> Vector Concatenate2/3
  Vector Concatenate2/1 -> Manual Switch/2
  C_B_N/1 -> Matrix Multiply/1  "c_B_N"
  Matrix Multiply/1 -> Sum/2
  Aero Forces/1 -> Manual Switch/1
  Manual Switch/1 -> Sum/1
  Initial Body Velocity/1 -> Integrator/2
  Accelerometer/1(Measured Acceleration) -> Manual Switch1/1  "measured Vdot_B_E_B"
  Manual Switch1/1 -> Integrator/1

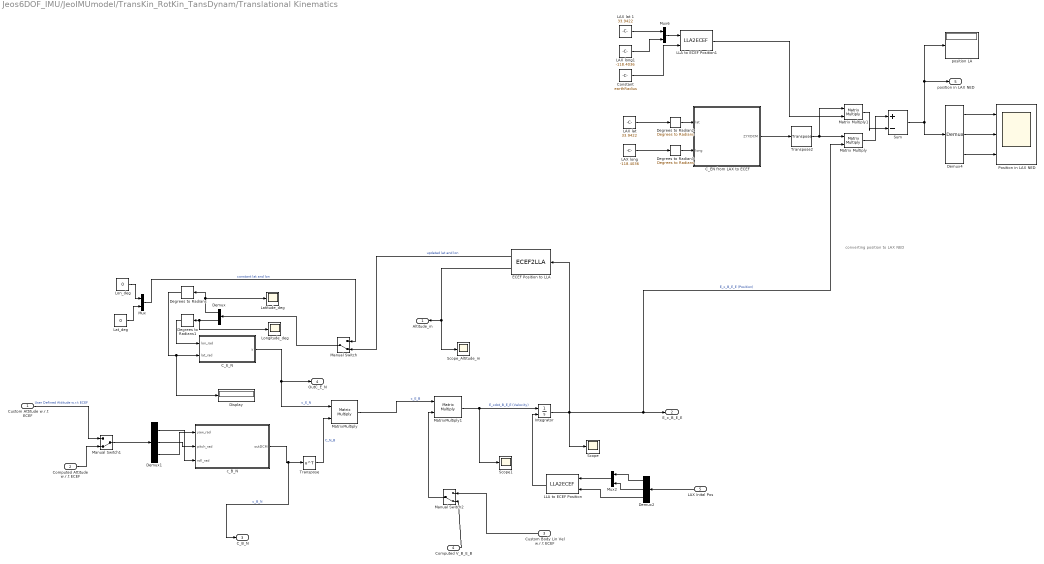
== system Jeos6DOF_IMU/JeoIMUmodel/TransKin_RotKin_TansDynam/Translational Kinematics ==
  note: converting position to LAX NED
  Custom Attitude w.r.t ECEF : Inport
  Computed Attitude w.r.t ECEF : Inport  Port=2
  Custom Body Lin Vel w.r.t ECEF : Inport  Port=3
  Computed V_B_E_B : Inport  Port=4
  LAX Inital Pos : Inport  Port=5
  C_EN from LAX to ECEF : MATLAB Function  TreatAsAtomicUnit=on
  C_E_N : MATLAB Function  TreatAsAtomicUnit=on
  Constant : Constant  Value=earthRadius
  Degrees to Radian2 : simulink_extras/Transformations/Degrees to Radians
  Degrees to Radian3 : simulink_extras/Transformations/Degrees to Radians
  Degrees to Radians : simulink_extras/Transformations/Degrees to Radians
  Degrees to Radians1 : simulink_extras/Transformations/Degrees to Radians
  Demux : Demux  Outputs=2
  Demux1 : Demux  Outputs=3
  Demux2 : Demux  Outputs=3
  Demux4 : Demux  Outputs=3
  Display : Display
  ECEF Position to LLA : ECEF2LLA  ptype=Custom
  Integrator : Integrator  InitialConditionSource=external  InitialCondition=[0;0;rEarth]
  "LAX lat " : Constant  Value=33.9422
  LAX lat 1 : Constant  Value=33.9422
  LAX long : Constant  Value=-118.4036
  LAX long1 : Constant  Value=-118.4036
  LLA to ECEF Position : LLA2ECEF  ptype=Custom
  LLA to ECEF Position1 : LLA2ECEF
  Lat_deg : Constant  Value=0
  Latitude_deg : Scope
  Lon_deg : Constant  Value=0
  Longitude_deg : Scope
  Manual Switch : ManualSwitch  CurrentSetting=0
  Manual Switch1 : ManualSwitch  CurrentSetting=0
  Manual Switch2 : ManualSwitch  CurrentSetting=0
  Matrix Multiply : Product  Multiplication=Matrix(*)
  Matrix Multiply1 : Product  Multiplication=Matrix(*)
  MatrixMultiply : Product  Multiplication=Matrix(*)
  MatrixMultiply1 : Product  Multiplication=Matrix(*)
  Mux : Mux  Inputs=2
  Mux2 : Mux  Inputs=2
  Mux6 : Mux  Inputs=2
  Position in LAX NED : Scope  NumInputPorts=3
  Scope : Scope
  Scope1 : Scope
  Scope_Altitude_m : Scope
  Sum : Sum  Inputs=|+-
  Transpose : Math  Operator=transpose
  Transpose2 : matrix_library/Transpose
  c_B_N : MATLAB Function  TreatAsAtomicUnit=on
  "position LA " : Display
  Altitude_m : Outport
  E_x_B_E_E : Outport  Port=2
  C_B_N : Outport  Port=3
  OutC_E_N : Outport  Port=4
  position in LAX NED : Outport  Port=5
  wires:
  MatrixMultiply1/1 -> Scope1/1, Integrator/1  "E_xdot_B_E_E (Velocity)"
  C_E_N/1(y) -> OutC_E_N/1, MatrixMultiply/1  "c_E_N"
  Manual Switch1/1 -> Demux1/1
  MatrixMultiply/1 -> MatrixMultiply1/1  "c_E_B"
  Degrees to Radians/1 -> Display/1, C_E_N/2(lat_rad)
  ECEF Position to LLA/2 -> Altitude_m/1, Scope_Altitude_m/1
  Transpose/1 -> MatrixMultiply/2  "C_N_B"
  Lon_deg/1 -> Mux/1
  Mux/1 -> Manual Switch/1  "constant lat and lon"
  Lat_deg/1 -> Mux/2
  Integrator/1 -> ECEF Position to LLA/1, Matrix Multiply/2, E_x_B_E_E/1, Scope/1  "E_x_B_E_E (Position)"
  ECEF Position to LLA/1 -> Manual Switch/2  "updated lat and lon"
  Demux1/3 -> c_B_N/1(yaw_rad)
  Demux1/1 -> c_B_N/3(roll_rad)
  Demux1/2 -> c_B_N/2(pitch_rad)
  c_B_N/1(outDCM) -> C_B_N/1, Transpose/1  "c_B_N"
  Manual Switch/1 -> Demux/1
  Manual Switch2/1 -> MatrixMultiply1/2
  Custom Attitude w.r.t ECEF/1 -> Manual Switch1/1  "User Defined Attitude w.r.t ECEF"
  Computed Attitude w.r.t ECEF/1 -> Manual Switch1/2
  Custom Body Lin Vel w.r.t ECEF/1 -> Manual Switch2/1
  Computed V_B_E_B/1 -> Manual Switch2/2
  Demux/2 -> Longitude_deg/1, Degrees to Radians1/1
  Demux/1 -> Degrees to Radians/1, Latitude_deg/1
  Degrees to Radians1/1 -> C_E_N/1(lon_rad)
  LAX Inital Pos/1 -> Demux2/1
  Demux2/1 -> Mux2/1
  Demux2/2 -> Mux2/2
  Demux2/3 -> LLA to ECEF Position/2
  Mux2/1 -> LLA to ECEF Position/1
  LLA to ECEF Position/1 -> Integrator/2
  LLA to ECEF Position1/1 -> Matrix Multiply1/2
  LAX long1/1 -> Mux6/2
  Matrix Multiply/1 -> Sum/1
  Demux4/2 -> Position in LAX NED/2
  Mux6/1 -> LLA to ECEF Position1/1
  Matrix Multiply1/1 -> Sum/2
  Constant/1 -> LLA to ECEF Position1/2
  LAX lat 1/1 -> Mux6/1
  Demux4/3 -> Position in LAX NED/3
  Demux4/1 -> Position in LAX NED/1
  C_EN from LAX to ECEF/1(ZYXDCM) -> Transpose2/1
  "LAX lat "/1 -> Degrees to Radian2/1
  Transpose2/1 -> Matrix Multiply1/1, Matrix Multiply/1
  LAX long/1 -> Degrees to Radian3/1
  Degrees to Radian2/1 -> C_EN from LAX to ECEF/1(lat)
  Degrees to Radian3/1 -> C_EN from LAX to ECEF/2(long)
  Sum/1 -> "position LA "/1, position in LAX NED/1, Demux4/1

== system Jeos6DOF_IMU/JeoIMUmodel/Aero Forces and Moments/F&M Horiz Stab Surface (S2)/F&M in Body ==
  momSurf : Inport
  Lift : Inport  Port=2
  Drag : Inport  Port=3
  v_B_E_B : Inport  Port=4
  n_s2 : Inport  Port=5
  Constant : Constant  Value=x_S2_B_B
  Force Due to Lift and Drag : MATLAB Function  TreatAsAtomicUnit=on
  Moment S2 : MATLAB Function  TreatAsAtomicUnit=on
  momS2_B : Outport
  LiftAndDragForceS2_B : Outport  Port=2
  wires:
  momSurf/1 -> Moment S2/1(momSurf)
  Lift/1 -> Force Due to Lift and Drag/1(lift)
  Drag/1 -> Force Due to Lift and Drag/2(drag)
  Force Due to Lift and Drag/1(forceLiftDragS2_B) -> Moment S2/2(FliftdragS), LiftAndDragForceS2_B/1
  v_B_E_B/1 -> Force Due to Lift and Drag/3(v_B_E_B)
  Moment S2/1(momS2_B) -> momS2_B/1
  n_s2/1 -> Force Due to Lift and Drag/4(n_s2), Moment S2/3(n_s2)
  Constant/1 -> Moment S2/4(x_S2_B_B)

== system Jeos6DOF_IMU/JeoIMUmodel/Aero Forces and Moments/F&M Horiz Stab Surface (S3)/F&M in Body ==
  momSurf : Inport
  Lift : Inport  Port=2
  Drag : Inport  Port=3
  v_B_E_B : Inport  Port=4
  n_s3 : Inport  Port=5
  Constant : Constant  Value=x_S3_B_B
  Force Due to Lift and Drag : MATLAB Function  TreatAsAtomicUnit=on
  Moment S3 : MATLAB Function  TreatAsAtomicUnit=on
  momS3_B : Outport
  LiftAndDragForceS3_B : Outport  Port=2
  wires:
  momSurf/1 -> Moment S3/1(momSurf)
  Lift/1 -> Force Due to Lift and Drag/1(lift)
  Drag/1 -> Force Due to Lift and Drag/2(drag)
  Force Due to Lift and Drag/1(forceLiftDragS3_B) -> Moment S3/2(FliftdragS), LiftAndDragForceS3_B/1
  v_B_E_B/1 -> Force Due to Lift and Drag/3(v_B_E_B)
  Moment S3/1(momS3_B) -> momS3_B/1
  n_s3/1 -> Force Due to Lift and Drag/4(n_s3), Moment S3/3(n_s3)
  Constant/1 -> Moment S3/4(x_S3_B_B)

== system Jeos6DOF_IMU/JeoIMUmodel/Aero Forces and Moments/F&M Right Wing and Servo Surface (S4)/F&M in Body ==
  momSurf : Inport
  Lift : Inport  Port=2
  Drag : Inport  Port=3
  v_B_E_B : Inport  Port=4
  n_s4 : Inport  Port=5
  Constant : Constant  Value=x_S4_B_B
  Force Due to Lift and Drag : MATLAB Function  TreatAsAtomicUnit=on
  Moment S4 : MATLAB Function  TreatAsAtomicUnit=on
  momS4_B : Outport
  LiftAndDragForceS4_B : Outport  Port=2
  wires:
  momSurf/1 -> Moment S4/1(momSurf)
  Lift/1 -> Force Due to Lift and Drag/1(lift)
  Drag/1 -> Force Due to Lift and Drag/2(drag)
  Force Due to Lift and Drag/1(forceLiftDragS4_B) -> Moment S4/2(FliftdragS), LiftAndDragForceS4_B/1
  v_B_E_B/1 -> Force Due to Lift and Drag/3(v_B_E_B)
  Moment S4/1(momS4_B) -> momS4_B/1
  n_s4/1 -> Force Due to Lift and Drag/4(n_s4), Moment S4/3(n_s4)
  Constant/1 -> Moment S4/4(x_S4_B_B)

== system Jeos6DOF_IMU/JeoIMUmodel/Aero Forces and Moments/F&M Right Wing and Servo Surface (S5)/F&M in Body ==
  momSurf : Inport
  Lift : Inport  Port=2
  Drag : Inport  Port=3
  v_B_E_B : Inport  Port=4
  n_s5 : Inport  Port=5
  Constant : Constant  Value=x_S5_B_B
  Force Due to Lift and Drag : MATLAB Function  TreatAsAtomicUnit=on
  Moment S5 : MATLAB Function  TreatAsAtomicUnit=on
  momS5_B : Outport
  LiftAndDragForceS5_B : Outport  Port=2
  wires:
  momSurf/1 -> Moment S5/1(momSurf)
  Lift/1 -> Force Due to Lift and Drag/1(lift)
  Drag/1 -> Force Due to Lift and Drag/2(drag)
  Force Due to Lift and Drag/1(forceLiftDragS5_B) -> Moment S5/2(FliftdragS), LiftAndDragForceS5_B/1
  v_B_E_B/1 -> Force Due to Lift and Drag/3(v_B_E_B)
  Moment S5/1(momS5_B) -> momS5_B/1
  n_s5/1 -> Force Due to Lift and Drag/4(n_s5), Moment S5/3(n_s5)
  Constant/1 -> Moment S5/4(x_S5_B_B)

== system Jeos6DOF_IMU/JeoIMUmodel/TransKin_RotKin_TansDynam/Translational Dynamics/Accelerometer ==
  True Acceleration : Inport
  Band-Limited White Noise : simulink/Sources/Band-Limited White Noise  Cov=[0.000001]  Ts=0.1  seed=[23341]
  Bias : Constant  Value=[0.025*9.8 0.025*9.8 0.025*9.8]
  Scale Factor : Gain  Gain=0.001
  Sum : Sum  Inputs=|++
  Sum1 : Sum  Inputs=|++
  Measured Acceleration : Outport
  wires:
  True Acceleration/1 -> Sum/1
  Bias/1 -> Sum/2
  Sum/1 -> Scale Factor/1
  Scale Factor/1 -> Sum1/1
  Band-Limited White Noise/1 -> Sum1/2
  Sum1/1 -> Measured Acceleration/1

== matlab function Jeos6DOF_IMU/JeoIMUmodel/Aero Forces and Moments/F&M Horiz Stab Surface (S2)/Compute Aero Moment ==
  data: v_B_E_B input; momSurf output; alphaLocal input; CM0_s2 input; CMa_s2 input; ro input; area_s2 input; c_s2 input
function momSurf = fcn(v_B_E_B, alphaLocal, CM0_s2, CMa_s2, ro, area_s2, c_s2)
% Compute the Moment at the respective Surface
% v_infSurf -> total airspeed at the surface, i.e. Velocity of body w.r.t Inertial/ECEF as
% measured in body frame (|V_B_E_B|)
% ro -> air density (note: varies with altitude)
% chordSurf -> Chord of the surface area
% cSurfM0 -> Initial moment coefficient of surface
% cSurfMalpha -> Moment coefficient at the respective surface due to the
% local alpha (Angle of Attack)
v_infSurf = norm(v_B_E_B);
cSurfMom = CM0_s2 + CMa_s2*alphaLocal; % Moment coefficient of surface
momSurf = cSurfMom * 0.5 * ro * (v_infSurf^2)*area_s2 * c_s2;

== matlab function Jeos6DOF_IMU/JeoIMUmodel/Aero Forces and Moments/F&M Horiz Stab Surface (S2)/F&M in Body/Force Due to Lift and Drag ==
  data: lift input; forceLiftDragS2_B output; drag input; v_B_E_B input; n_s2 input
function forceLiftDragS2_B = fcn(lift, drag, v_B_E_B, n_s2)

forceLiftDrag_w = lift*n_s2 - [drag; 0; 0];
alpha = atan2(v_B_E_B(3), v_B_E_B(1));
beta = asin(v_B_E_B(2) / norm(v_B_E_B));

c_S_B = [cos(alpha), 0, sin(alpha); 0, 1, 0; -sin(alpha), 0, cos(alpha)] ;
c_W_S = [cos(beta), sin(beta), 0; -sin(beta), cos(beta), 0; 0,0,1];
c_W_B = c_W_S * c_S_B;

forceLiftDragS2_B = c_W_B' * forceLiftDrag_w;

== matlab function Jeos6DOF_IMU/JeoIMUmodel/Aero Forces and Moments/F&M Right Wing and Servo Surface (S4)/Compute Aero Lift and Drag ==
  data: v_B_E_B input; alphaLocal output; v_B_A_B input; liftSurf output; dragSurf output; AR_s4 input; i_s4 input; n_s4 input; CL0_s4 input; CD0_s4 input; CDa_s4 input; a0_s4 input; e_s4 input; ro input; area_s4 input
function [alphaLocal, liftSurf, dragSurf] = fcn(v_B_E_B, v_B_A_B, AR_s4, i_s4, n_s4, CL0_s4, CD0_s4, CDa_s4, a0_s4, e_s4, ro, area_s4)
% Compute the lift and drag forces at the respective surface
% arSurf -> Aspect Ratio of respective surfaace
% ro -> air density (note: varies with altitude)
% v_infSurf -> total airspeed at the surface, i.e. Velocity of body w.r.t Inertial/ECEF as
% measured in body frame (|V_B_E_B|)
% v_B_A_B -> relative airspeed, where it is typically 
% v_B_E_B - c_B_N * v_A_N_N and v_A_N_N is the velocity of air mass w.r.t. NED 
% nSurf_B -> Normal force applied at surface
% eSurf -> Oswald efficiency
% alphaLocal0 -> Minimum drag Angle of Attack

v_infSurf = norm(v_B_E_B);
cSurfLocAlpha = 2*pi * (AR_s4/(2+AR_s4)); % Lift coefficient at the respective surface due to the local alpha (Angle of Attack)
alphaLocal = i_s4 - asin(dot(v_B_A_B,n_s4)/norm(v_B_A_B)); % in Radians
cSurfLift = CL0_s4 + cSurfLocAlpha * alphaLocal; % Lift coefficient of surface
cSurfDrag = CD0_s4 + CDa_s4 *(alphaLocal - a0_s4)^2 + (cSurfLift^2/(pi*e_s4*AR_s4));

liftSurf = cSurfLift * 0.5 * ro * (v_infSurf^2)*area_s4;
dragSurf = cSurfDrag * 0.5 * ro * (v_infSurf^2)*area_s4;

== matlab function Jeos6DOF_IMU/JeoIMUmodel/Aero Forces and Moments/F&M Right Wing and Servo Surface (S4)/Compute Aero Moment ==
  data: v_B_E_B input; momSurf output; alphaLocal input; CM0_s4 input; CMa_s4 input; ro input; area_s4 input; c_s4 input
function momSurf = fcn(v_B_E_B, alphaLocal, CM0_s4, CMa_s4, ro, area_s4, c_s4)
% Compute the Moment at the respective Surface
% v_infSurf -> total airspeed at the surface, i.e. Velocity of body w.r.t Inertial/ECEF as
% measured in body frame (|V_B_E_B|)
% ro -> air density (note: varies with altitude)
% chordSurf -> Chord of the surface area
% cSurfM0 -> Initial moment coefficient of surface
% cSurfMalpha -> Moment coefficient at the respective surface due to the
% local alpha (Angle of Attack)
v_infSurf = norm(v_B_E_B);
cSurfMom = CM0_s4 + CMa_s4*alphaLocal; % Moment coefficient of surface
momSurf = cSurfMom * 0.5 * ro * (v_infSurf^2)*area_s4 * c_s4;

== matlab function Jeos6DOF_IMU/JeoIMUmodel/Aero Forces and Moments/F&M Right Wing and Servo Surface (S4)/F&M in Body/Force Due to Lift and Drag ==
  data: lift input; forceLiftDragS4_B output; drag input; v_B_E_B input; n_s4 input
function forceLiftDragS4_B = fcn(lift, drag, v_B_E_B, n_s4)

forceLiftDrag_w = lift*n_s4 - [drag; 0; 0];
alpha = atan2(v_B_E_B(3), v_B_E_B(1));
beta = asin(v_B_E_B(2) / norm(v_B_E_B));

c_S_B = [cos(alpha), 0, sin(alpha); 0, 1, 0; -sin(alpha), 0, cos(alpha)] ;
c_W_S = [cos(beta), sin(beta), 0; -sin(beta), cos(beta), 0; 0,0,1];
c_W_B = c_W_S * c_S_B;

forceLiftDragS4_B = c_W_B' * forceLiftDrag_w;

== matlab function Jeos6DOF_IMU/JeoIMUmodel/Aero Forces and Moments/F&M Right Wing and Servo Surface (S4)/F&M in Body/Moment S4 ==
  data: momSurf input; momS4_B output; FliftdragS input; n_s4 input; x_S4_B_B input
function momS4_B = fcn(momSurf, FliftdragS, n_s4, x_S4_B_B)
% Compute the moment at the respective surface
crot = [0,0,0; 0,0,-1; 0,1,0];

momS4_B = momSurf * crot* n_s4 + (cross(x_S4_B_B, FliftdragS));

== matlab function Jeos6DOF_IMU/JeoIMUmodel/Aero Forces and Moments/F&M Right Wing and Servo Surface (S5)/Compute Aero Lift and Drag ==
  data: v_B_E_B input; alphaLocal output; v_B_A_B input; liftSurf output; dragSurf output; AR_s5 input; i_s5 input; n_s5 input; CL0_s5 input; CD0_s5 input; CDa_s5 input; a0_s5 input; e_s5 input; ro input; area_s5 input
function [alphaLocal, liftSurf, dragSurf] = fcn(v_B_E_B, v_B_A_B, AR_s5, i_s5, n_s5, CL0_s5, CD0_s5, CDa_s5, a0_s5, e_s5, ro, area_s5)
% Compute the lift and drag forces at the respective surface
% arSurf -> Aspect Ratio of respective surfaace
% ro -> air density (note: varies with altitude)
% v_infSurf -> total airspeed at the surface, i.e. Velocity of body w.r.t Inertial/ECEF as
% measured in body frame (|V_B_E_B|)
% v_B_A_B -> relative airspeed, where it is typically 
% v_B_E_B - c_B_N * v_A_N_N and v_A_N_N is the velocity of air mass w.r.t. NED 
% nSurf_B -> Normal force applied at surface
% eSurf -> Oswald efficiency
% alphaLocal0 -> Minimum drag Angle of Attack

v_infSurf = norm(v_B_E_B);
cSurfLocAlpha = 2*pi * (AR_s5/(2+AR_s5)); % Lift coefficient at the respective surface due to the local alpha (Angle of Attack)
alphaLocal = i_s5 - asin(dot(v_B_A_B,n_s5)/norm(v_B_A_B)); % in Radians
cSurfLift = CL0_s5 + cSurfLocAlpha * alphaLocal; % Lift coefficient of surface
cSurfDrag = CD0_s5 + CDa_s5 *(alphaLocal - a0_s5)^2 + (cSurfLift^2/(pi*e_s5*AR_s5));

liftSurf = cSurfLift * 0.5 * ro * (v_infSurf^2)*area_s5;
dragSurf = cSurfDrag * 0.5 * ro * (v_infSurf^2)*area_s5;

== matlab function Jeos6DOF_IMU/JeoIMUmodel/TransKin_RotKin_TansDynam/Translational Kinematics/c_B_N ==
  data: yaw_rad input; outDCM output; pitch_rad input; roll_rad input
function outDCM = euler2DCM_TB(yaw_rad, pitch_rad, roll_rad)
% This functions takes in yaw, pitch and roll angles to compute the
% Tait-Bryan ZYX sequence DCM from reference frame (NED) to Body Frame
yawDCM = [cos(yaw_rad), sin(yaw_rad), 0; -sin(yaw_rad), cos(yaw_rad), 0; 0, 0, 1];
pitchDCM = [cos(pitch_rad), 0, -sin(pitch_rad); 0, 1, 0; sin(pitch_rad), 0, cos(pitch_rad)];

rollDCM = [1,0,0; 0, cos(roll_rad), sin(roll_rad); 0, -sin(roll_rad), cos(roll_rad)];
%outDCM = yawDCM*pitchDCM*rollDCM;
outDCM = rollDCM*pitchDCM*yawDCM;
end

== matlab function Jeos6DOF_IMU/JeoIMUmodel/Aero Forces and Moments/F&M Right Wing and Servo Surface (S5)/Compute Aero Moment ==
  data: v_B_E_B input; momSurf output; alphaLocal input; CM0_s5 input; CMa_s5 input; ro input; area_s5 input; c_s5 input
function momSurf = fcn(v_B_E_B, alphaLocal, CM0_s5, CMa_s5, ro, area_s5, c_s5)
% Compute the Moment at the respective Surface
% v_infSurf -> total airspeed at the surface, i.e. Velocity of body w.r.t Inertial/ECEF as
% measured in body frame (|V_B_E_B|)
% ro -> air density (note: varies with altitude)
% chordSurf -> Chord of the surface area
% cSurfM0 -> Initial moment coefficient of surface
% cSurfMalpha -> Moment coefficient at the respective surface due to the
% local alpha (Angle of Attack)
v_infSurf = norm(v_B_E_B);
cSurfMom = CM0_s5 + CMa_s5*alphaLocal; % Moment coefficient of surface
momSurf = cSurfMom * 0.5 * ro * (v_infSurf^2)*area_s5 * c_s5;

== matlab function Jeos6DOF_IMU/JeoIMUmodel/Aero Forces and Moments/F&M Right Wing and Servo Surface (S5)/F&M in Body/Force Due to Lift and Drag ==
  data: lift input; forceLiftDragS5_B output; drag input; v_B_E_B input; n_s5 input
function forceLiftDragS5_B = fcn(lift, drag, v_B_E_B, n_s5)

forceLiftDrag_w = lift*n_s5 - [drag; 0; 0];
alpha = atan2(v_B_E_B(3), v_B_E_B(1));
beta = asin(v_B_E_B(2) / norm(v_B_E_B));

c_S_B = [cos(alpha), 0, sin(alpha); 0, 1, 0; -sin(alpha), 0, cos(alpha)] ;
c_W_S = [cos(beta), sin(beta), 0; -sin(beta), cos(beta), 0; 0,0,1];
c_W_B = c_W_S * c_S_B;

forceLiftDragS5_B = c_W_B' * forceLiftDrag_w;

== matlab function Jeos6DOF_IMU/JeoIMUmodel/Aero Forces and Moments/F&M Right Wing and Servo Surface (S5)/F&M in Body/Moment S5 ==
  data: momSurf input; momS5_B output; FliftdragS input; n_s5 input; x_S5_B_B input
function momS5_B = fcn(momSurf, FliftdragS, n_s5, x_S5_B_B)
% Compute the moment at the respective surface
crot = [0,0,0; 0,0,-1; 0,1,0];

momS5_B = momSurf * crot* n_s5 + (cross(x_S5_B_B, FliftdragS));

== matlab function Jeos6DOF_IMU/JeoIMUmodel/Aero Forces and Moments/F&M Horiz Stab Surface (S2)/F&M in Body/Moment S2 ==
  data: momSurf input; momS2_B output; FliftdragS input; n_s2 input; x_S2_B_B input
function momS2_B = fcn(momSurf, FliftdragS, n_s2, x_S2_B_B)
% Compute the moment at the respective surface
crot = [0,0,0; 0,0,-1; 0,1,0];

momS2_B = momSurf * crot* n_s2 + (cross(x_S2_B_B, FliftdragS));

== matlab function Jeos6DOF_IMU/JeoIMUmodel/Aero Forces and Moments/F&M Horiz Stab Surface (S3)/Compute Aero Lift and Drag ==
  data: v_B_E_B input; alphaLocal output; v_B_A_B input; liftSurf output; dragSurf output; AR_s3 input; i_s3 input; n_s3 input; CL0_s3 input; CD0_s3 input; CDa_s3 input; a0_s3 input; e_s3 input; ro input; area_s3 input
function [alphaLocal, liftSurf, dragSurf] = fcn(v_B_E_B, v_B_A_B, AR_s3, i_s3, n_s3, CL0_s3, CD0_s3, CDa_s3, a0_s3, e_s3, ro, area_s3)
% Compute the lift and drag forces at the respective surface
% arSurf -> Aspect Ratio of respective surfaace
% ro -> air density (note: varies with altitude)
% v_infSurf -> total airspeed at the surface, i.e. Velocity of body w.r.t Inertial/ECEF as
% measured in body frame (|V_B_E_B|)
% v_B_A_B -> relative airspeed, where it is typically 
% v_B_E_B - c_B_N * v_A_N_N and v_A_N_N is the velocity of air mass w.r.t. NED 
% nSurf_B -> Normal force applied at surface
% eSurf -> Oswald efficiency
% alphaLocal0 -> Minimum drag Angle of Attack

v_infSurf = norm(v_B_E_B);
cSurfLocAlpha = 2*pi * (AR_s3/(2+AR_s3)); % Lift coefficient at the respective surface due to the local alpha (Angle of Attack)
alphaLocal = i_s3 - asin(dot(v_B_A_B,n_s3)/norm(v_B_A_B)); % in Radians
cSurfLift = CL0_s3 + cSurfLocAlpha * alphaLocal; % Lift coefficient of surface
cSurfDrag = CD0_s3 + CDa_s3 *(alphaLocal - a0_s3)^2 + (cSurfLift^2/(pi*e_s3*AR_s3));

liftSurf = cSurfLift * 0.5 * ro * (v_infSurf^2)*area_s3;
dragSurf = cSurfDrag * 0.5 * ro * (v_infSurf^2)*area_s3;

== matlab function Jeos6DOF_IMU/JeoIMUmodel/Aero Forces and Moments/F&M Horiz Stab Surface (S3)/Compute Aero Moment ==
  data: v_B_E_B input; momSurf output; alphaLocal input; CM0_s3 input; CMa_s3 input; ro input; area_s3 input; c_s3 input
function momSurf = fcn(v_B_E_B, alphaLocal, CM0_s3, CMa_s3, ro, area_s3, c_s3)
% Compute the Moment at the respective Surface
% v_infSurf -> total airspeed at the surface, i.e. Velocity of body w.r.t Inertial/ECEF as
% measured in body frame (|V_B_E_B|)
% ro -> air density (note: varies with altitude)
% chordSurf -> Chord of the surface area
% cSurfM0 -> Initial moment coefficient of surface
% cSurfMalpha -> Moment coefficient at the respective surface due to the
% local alpha (Angle of Attack)
v_infSurf = norm(v_B_E_B);
cSurfMom = CM0_s3 + CMa_s3*alphaLocal; % Moment coefficient of surface
momSurf = cSurfMom * 0.5 * ro * (v_infSurf^2)*area_s3 * c_s3;

== matlab function Jeos6DOF_IMU/JeoIMUmodel/Aero Forces and Moments/F&M Horiz Stab Surface (S3)/F&M in Body/Force Due to Lift and Drag ==
  data: lift input; forceLiftDragS3_B output; drag input; v_B_E_B input; n_s3 input
function forceLiftDragS3_B = fcn(lift, drag, v_B_E_B, n_s3)

forceLiftDrag_w = lift*n_s3 - [drag; 0; 0];
alpha = atan2(v_B_E_B(3), v_B_E_B(1));
beta = asin(v_B_E_B(2) / norm(v_B_E_B));

c_S_B = [cos(alpha), 0, sin(alpha); 0, 1, 0; -sin(alpha), 0, cos(alpha)] ;
c_W_S = [cos(beta), sin(beta), 0; -sin(beta), cos(beta), 0; 0,0,1];
c_W_B = c_W_S * c_S_B;

forceLiftDragS3_B = c_W_B' * forceLiftDrag_w;

== matlab function Jeos6DOF_IMU/JeoIMUmodel/TransKin_RotKin_TansDynam/Translational Kinematics/C_E_N ==
  data: lon_rad input; y output; lat_rad input
function y = NEDtoECEF(lon_rad, lat_rad)
% DCM to go from NED to ECEF frame

firstRot = [cos(lon_rad), cos(lon_rad), 0; -sin(lon_rad), cos(lon_rad), 0; 0, 0, 1;]; % Rotate about longitude first

secondRot = [0, 0, 1; 0, 1, 0; -1, 0,0]; % Left handed rotation of 90 deg 

thirdRot = [cos(lat_rad),0,sin(lat_rad); 0,1,0; -sin(lat_rad), 0, cos(lat_rad)];
% Multiply to get ECEF to NED DCM

c_NED_ECEF = thirdRot*secondRot*firstRot;
y = c_NED_ECEF';

== matlab function Jeos6DOF_IMU/JeoIMUmodel/Aero Forces and Moments/F&M Horiz Stab Surface (S3)/F&M in Body/Moment S3 ==
  data: momSurf input; momS3_B output; FliftdragS input; n_s3 input; x_S3_B_B input
function momS3_B = fcn(momSurf, FliftdragS, n_s3, x_S3_B_B)
% Compute the moment at the respective surface
crot = [0,0,0; 0,0,-1; 0,1,0];

momS3_B = momSurf * crot* n_s3 + (cross(x_S3_B_B, FliftdragS));
